simulink model "s_c856m4k"  (R2016b)
(part 3 of 92)

  Subsystem2/1(out0) -> cd_status/1(out_pol0_err_cnt)
  cd_compensation1/4(hmc_error) -> [cd_error_p1]
  [cd_error_p0] -> pipeline146/1(d)
  [cd_error_p1] -> pipeline147/1(d)
  pipeline146/1(q) -> snap_cd_time_debug/10(in_cd_error0)
  pipeline147/1(q) -> snap_cd_time_debug/11(in_cd_error1)
